simulink model "questao01_1_final_well"  (R2020a)
settings: Solver=VariableStepAuto  StartTime=0.0  StopTime=20  RelTol=1e-3
values from neighbouring files (symbols this model uses):
  A = [1 2 0;-1 -1 -1;0 2 -1]    [lqr_estudos.m]    (also in questao2_pat.m = [1 2 0; -1 -1 -1; 0 2 -1])
  B = [0;0;2]    [lqr_estudos.m]    (also in questao2_pat.m)
  C = [0 1 0;0 0 1]    [lqr_estudos.m]    (also in questao2_pat.m = [0 1 0; 0 0 1])
  K = place(A,B,poles)    [estudos_versao_laurinda.m]    (also in lqr_estudos.m = lqr(A,B,Q,R); questao1_pat.m = Ka(1:3); questao1_well.m = Ka(1:3); questao2_pat.m = place(A,B,newpoles))
  Kz = 1    [estudos_versao_laurinda.m]    (also in questao1_pat.m = Ka(4); questao1_well.m = Ka(4))
  L = L'    [questao1_pat.m]    (also in questao2_pat.m)
undefined symbols (not defined in the file or in its folder): sigbuilder_block
settings Model: Creator=wwagner  LastModifiedBy=wwagner

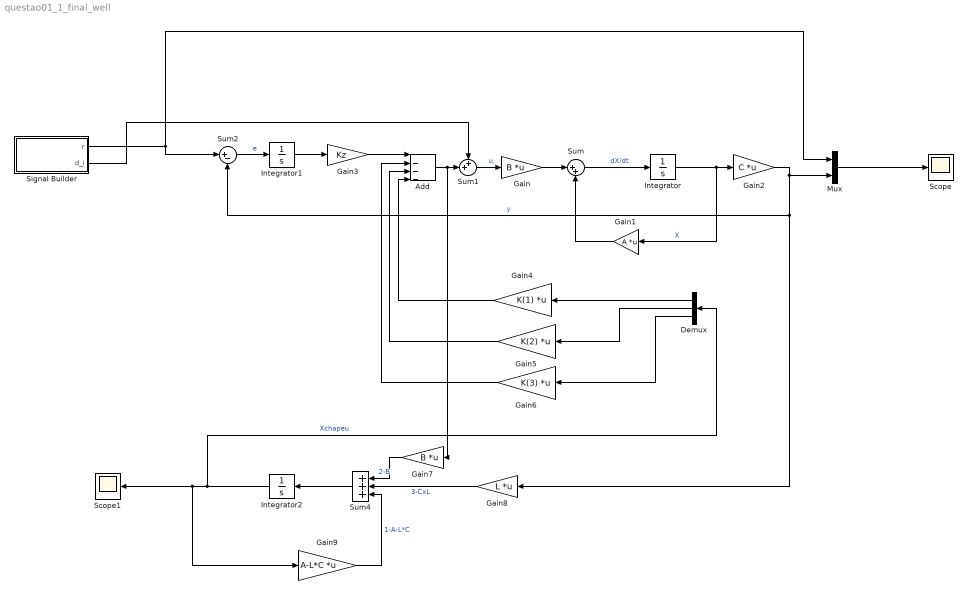
== system questao01_1_final_well ==
  Add : Sum  Inputs=----
  Demux : Demux  Outputs=3
  Gain : Gain  Gain=B  Multiplication=Matrix(K*u)
  Gain1 : Gain  Gain=A  Multiplication=Matrix(K*u)
  Gain2 : Gain  Gain=C  Multiplication=Matrix(K*u)
  Gain3 : Gain  Gain=Kz
  Gain4 : Gain  Gain=K(1)  Multiplication=Matrix(K*u)
  Gain5 : Gain  Gain=K(2)  Multiplication=Matrix(K*u)
  Gain6 : Gain  Gain=K(3)  Multiplication=Matrix(K*u)
  Gain7 : Gain  Gain=B  Multiplication=Matrix(K*u)
  Gain8 : Gain  Gain=L  Multiplication=Matrix(K*u)
  Gain9 : Gain  Gain=A-L*C  Multiplication=Matrix(K*u)
  Integrator : Integrator
  Integrator1 : Integrator
  Integrator2 : Integrator
  Mux : Mux  Inputs=2
  Scope : Scope
  Scope1 : Scope
  Signal Builder : Subsystem  Tag=STV Subsys  LoadFcn=sigbuilder_block('load');  StartFcn=sigbuilder_block('start');  StopFcn=sigbuilder_block('stop');  ClipboardFcn=sigbuilder_block('clipboard');  mask(Sigbuilder block){tuvar=[0:10]}
      mask help: Simulink:masks:SigbuilderBlock_MD
      mask init:
      | if ~strcmp(get_param(bdroot(gcbh),'SimulationStatus'),'stopped') tuvar = sigbuilder_block('maskInit'); end
      settings: CopyFcn=sigbuilder_block('copy');  DeleteFcn=sigbuilder_block('delete');  ModelCloseFcn=sigbuilder_block('modelClose');  PreSaveFcn=sigbuilder_block('preSave');  PauseFcn=sigbuilder_block('pause');  ContinueFcn=sigbuilder_block('continue');  NameChangeFcn=sigbuilder_block('namechange');  OpenFcn=sigbuilder_block('open',[299 204 690 436 ]);  CloseFcn=sigbuilder_block('close');
      mask Display: plot(0, 0, 100, 100,[2, 2, 32, 32, 2], [68, 8, 8, 68, 68],[32, 2], [38, 38], [32, 19, 2],[53, 60, 44], [32, 17, 17, 2],[16, 16, 31, 31]);txt = getActiveGroup(gcbh);text(2, 100, txt,'verticalAlignment', 'top');
  Sum : Sum  Inputs=|++
  Sum1 : Sum  Inputs=++|
  Sum2 : Sum  Inputs=|+-
  Sum4 : Sum  Inputs=+++
  wires:
  Integrator/1 -> Gain1/1, Gain2/1  "X"
  Gain/1 -> Sum/1
  Gain1/1 -> Sum/2
  Sum/1 -> Integrator/1  "dX/dt"
  Gain2/1 -> Mux/2, Gain8/1, Sum2/2  "y"
  Mux/1 -> Scope/1
  Sum2/1 -> Integrator1/1  "e"
  Integrator1/1 -> Gain3/1
  Demux/1 -> Gain4/1
  Demux/2 -> Gain5/1
  Demux/3 -> Gain6/1
  Gain3/1 -> Add/1
  Gain4/1 -> Add/4
  Gain5/1 -> Add/3
  Gain6/1 -> Add/2
  Sum1/1 -> Gain/1  "u"
  Add/1 -> Gain7/1, Sum1/2
  Gain7/1 -> Sum4/1  "2-B"
  Sum4/1 -> Integrator2/1
  Integrator2/1 -> Gain9/1, Scope1/1, Demux/1  "Xchapeu"
  Gain8/1 -> Sum4/2  "3-CxL"
  Gain9/1 -> Sum4/3  "1-A-L*C"
  Signal Builder/1(r) -> Sum2/1, Mux/1
  Signal Builder/2(d_i) -> Sum1/1

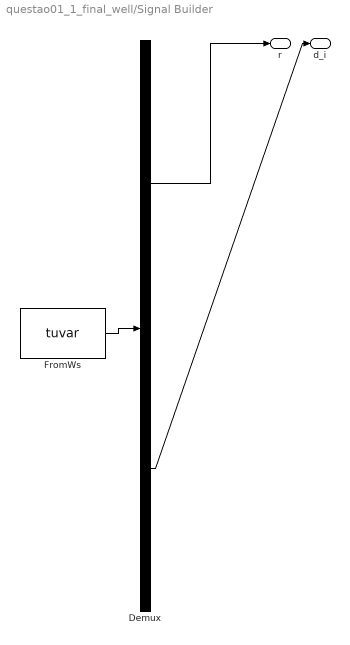
== system questao01_1_final_well/Signal Builder ==
  Demux : Demux  Tag=STV Demux  Outputs=2
      settings: DisplayOption=none
  FromWs : FromWorkspace  Tag=STV FromWs  VariableName=tuvar
      SigBuilderData=|
      | common.afterFinalStr = 'Extrapolate'
      | common.sampleTime = 0
      | dataSet.timeRange = [-10 20]
      | dataSet.name = 'Group 1'
      | sbobj.Groups.Name = 'Group 1'
      | sbobj.Groups.Signals(1).Name = 'r'
      | sbobj.Groups.Signals(1).XData = [-10 0 0 7.49 7.5 20]
      | sbobj.Groups.Signals(1).YData = [0 0 2 2 1 1]
      | sbobj.Groups.Signals(2).Name = 'd_i'
      | sbobj.Groups.Signals(2).XData = [-10 20]
      | sbobj.Groups.Signals(2).YData = [0 0]
      | sbobj.Groups.TimeRange = [-10 20]
  r : Outport  Tag=STV Outport
  d_i : Outport  Tag=STV Outport  Port=2
  wires:
  Demux/1 -> r/1
  FromWs/1 -> Demux/1
  Demux/2 -> d_i/1
